simulink library "magnetic_field_lib"  (R2016b)
settings: Solver=ode45  StartTime=0.0  StopTime=10.0  RelTol=1e-3  EnableMultiTasking=on
undefined symbols (not defined in the file or in its folder): Earth, sim_params, WGS84
libraries: aerolibtransform2 x2, aerolibgravity2 x1, vrlib x1
settings Model: Creator=bbarz_000  LastModifiedBy=taylorreynolds
settings DataIOCC: LimitDataPoints=on
settings OptimizationCC: LifeSpan=inf
settings DebuggingCC: AllowSymbolicDim=off  SFUnexpectedBacktrackingDiag=warning  SFNoUnconditionalDefaultTransitionDiag=warning  SFExecutionAtInitializationDiag=none
settings GRTTargetCC: TargetLangStandard=C89/C90 (ANSI)  GeneratePreprocessorConditionals=Disable all
settings ConfigComp: CovMetricSettings=dw  CovHtmlReporting=on  CovSaveCumulativeToWorkspaceVar=on  CovSaveSingleToWorkspaceVar=on  CovExternalEMLEnable=off

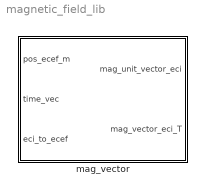
== system magnetic_field_lib ==
  mag_vector : Subsystem

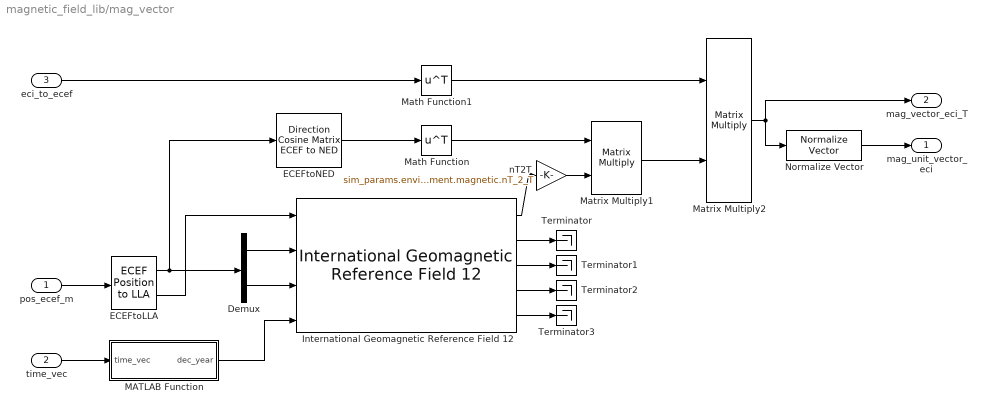
== system magnetic_field_lib/mag_vector ==
  pos_ecef_m : Inport
  time_vec : Inport  Port=2
  eci_to_ecef : Inport  Port=3
  Demux : Demux  Outputs=2
  ECEFtoLLA : aerolibtransform2/ECEF Position to LLA  units=Metric (MKS)  ptype=Earth (WGS84)  F=1/298.257223563  R=6378137
  ECEFtoNED : aerolibtransform2/Direction Cosine Matrix ECEF to NED
  International Geomagnetic Reference Field 12 : aerolibgravity2/International Geomagnetic Reference Field 12  units=Metric (MKS)  time_in=on  month=January  day=1  year=2020  action=None  sv_out=off
  MATLAB Function : MATLAB Function  TreatAsAtomicUnit=on
  Math Function : Math  Operator=transpose  SaturateOnIntegerOverflow=on
  Math Function1 : Math  Operator=transpose  SaturateOnIntegerOverflow=on
  Matrix Multiply1 : Product  Multiplication=Matrix(*)
  Matrix Multiply2 : Product  Multiplication=Matrix(*)
  Normalize Vector : vrlib/Utilities/Normalize Vector  maxzero=0
  Terminator{,1..3} (4 alike) : Terminator
  nT2T : Gain  Gain=sim_params.environment.magnetic.nT_2_T
  mag_unit_vector_eci : Outport
  mag_vector_eci_T : Outport  Port=2
  wires:
  pos_ecef_m/1 -> ECEFtoLLA/1
  Normalize Vector/1 -> mag_unit_vector_eci/1
  Matrix Multiply2/1 -> Normalize Vector/1, mag_vector_eci_T/1
  Matrix Multiply1/1 -> Matrix Multiply2/2
  Math Function1/1 -> Matrix Multiply2/1
  Math Function/1 -> Matrix Multiply1/1
  ECEFtoNED/1 -> Math Function/1
  time_vec/1 -> MATLAB Function/1(time_vec)
  nT2T/1 -> Matrix Multiply1/2
  International Geomagnetic Reference Field 12/1 -> nT2T/1
  Demux/2 -> International Geomagnetic Reference Field 12/3
  Demux/1 -> International Geomagnetic Reference Field 12/2
  ECEFtoLLA/1 -> Demux/1, ECEFtoNED/1
  eci_to_ecef/1 -> Math Function1/1
  ECEFtoLLA/2 -> International Geomagnetic Reference Field 12/1
  MATLAB Function/1(dec_year) -> International Geomagnetic Reference Field 12/4
  International Geomagnetic Reference Field 12/2 -> Terminator/1
  International Geomagnetic Reference Field 12/3 -> Terminator1/1
  International Geomagnetic Reference Field 12/4 -> Terminator2/1
  International Geomagnetic Reference Field 12/5 -> Terminator3/1

== matlab function magnetic_field_lib/mag_vector/MATLAB Function ==
  data: time_vec input size=6; dec_year output size=1
function dec_year = fcn(time_vec)

% UW HuskySat 1, ADCS Subsystem
%   T. Reynolds, Updated: 8.24.17

% Converts a time vector into a decimal year number. See Vallado pp 200-201
% for reference algorithms.

year    = time_vec(1);
month   = time_vec(2);
day     = time_vec(3);
hour    = time_vec(4);
min     = time_vec(5);
sec     = time_vec(6);

% find day of year - valid until 2100
Lmonth = [31, 28, 31, 30, 31, 30, 31, 31, 30, 31, 30, 31];
days_in_year    = 365.25;

if mod(year,4) == 0
    Lmonth(2) = 29;
    days_in_year    = 366;
end

day_of_year = 0;
for i = 1:month-1
    day_of_year = day_of_year + Lmonth(i);
end

% Add number of days into the month
day_of_year = day_of_year + day;

% Add HMS info to the day of year
day_of_year    = day_of_year + hour/24 + min/1440 + sec/86400;

% Find the year fraction represented by day_of_year
day_frac    = day_of_year/days_in_year;

% Sum to get total decimal year
dec_year = year + day_frac;


end
